simulink model "main"  (R2024b)
settings: Solver=FixedStepAuto  StartTime=0.0  StopTime=5  FixedStep=Ts  RelTol=1e-3
values from neighbouring files (symbols this model uses):
  v0 = 30    [main_data_vehicle.m]
settings Model: Creator=marti  LastModifiedBy=marti

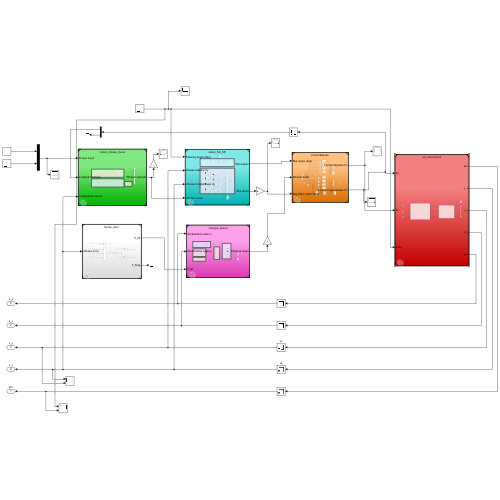
[thumbnail: Simulink's stored preview of the top-level diagram]
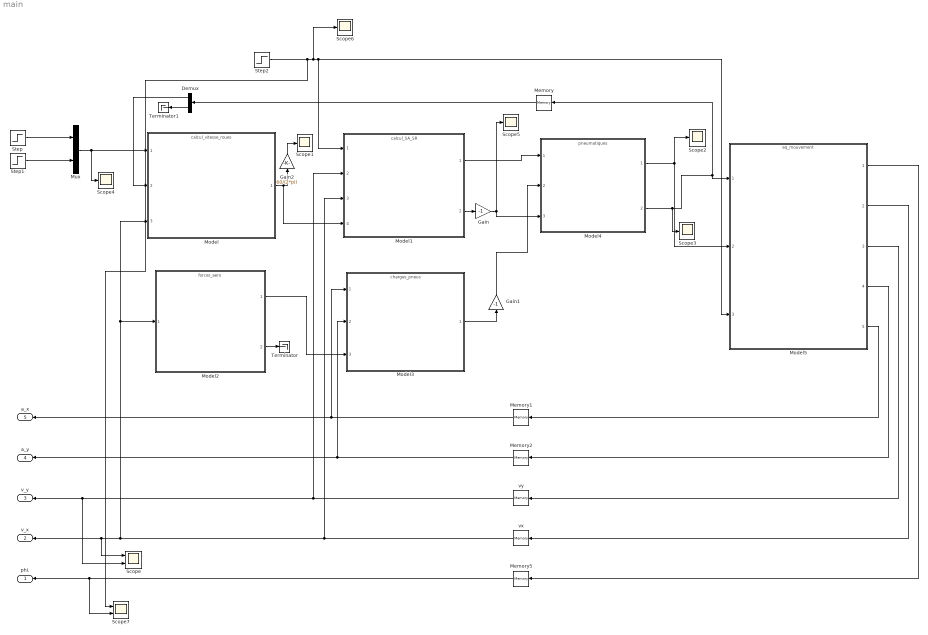
== system main ==
  Demux : Demux  Outputs=2
  Gain : Gain  Gain=-1
  Gain1 : Gain  Gain=-1
  Gain2 : Gain  Gain=60/(2*pi)
  Memory : Memory  InitialCondition=[0 0 0 0]
  Memory1 : Memory
  Memory2 : Memory
  Memory5 : Memory
  Model : ModelReference  ModelNameDialog=calcul_vitesse_roues.slx  SimulationMode=Normal  ModelReferenceVersion=1.19
  Model1 : ModelReference  ModelNameDialog=calcul_SA_SR.slx  SimulationMode=Normal  ModelReferenceVersion=1.19
  Model2 : ModelReference  ModelNameDialog=forces_aero.slx  SimulationMode=Normal  ModelReferenceVersion=1.4
  Model3 : ModelReference  ModelNameDialog=charges_pneus.slx  SimulationMode=Normal  ModelReferenceVersion=1.16
  Model4 : ModelReference  ModelNameDialog=pneumatiques.slx  SimulationMode=Normal  ModelReferenceVersion=1.15
  Model5 : ModelReference  ModelNameDialog=eq_mouvement.slx  SimulationMode=Normal  ModelReferenceVersion=1.6
  Mux : Mux  Inputs=2
  Scope : Scope  NumInputPorts=2
  Scope{1..6} (6 alike) : Scope
  Scope7 : Scope  NumInputPorts=2
  Step : Step  Time=0  After=100  SampleTime=0
  Step1 : Step  Time=0  After=300  SampleTime=0
  Step2 : Step  Time=0  After=0  SampleTime=0
  Terminator : Terminator
  Terminator1 : Terminator
  vx : Memory  InitialCondition=v0
  vy : Memory
  phi. : Outport
  v_x : Outport  Port=2
  v_y : Outport  Port=3
  a_y : Outport  Port=4
  a_x : Outport  Port=5
  wires:
  Model2/1 -> Model3/3
  Model2/2 -> Terminator/1
  Model/1 -> Model1/4, Gain2/1
  Model4/1 -> Scope2/1, Model5/2
  Model4/2 -> Scope3/1, Memory/1, Model5/1
  Model5/1 -> Memory5/1
  Model5/3 -> vy/1
  Model5/4 -> Memory2/1
  Model5/5 -> Memory1/1
  Model5/2 -> vx/1
  Step2/1 -> Scope7/1, Scope6/1, Model5/3, Model1/1
  Mux/1 -> Scope4/1, Model/1
  Memory/1 -> Demux/1
  Demux/1 -> Model/2
  Demux/2 -> Terminator1/1
  Memory1/1 -> Model3/1, a_x/1
  Memory2/1 -> Model3/2, a_y/1
  vy/1 -> Model1/2, Scope/2, v_y/1
  vx/1 -> Model1/3, Model/3, Model2/1, Scope/1, v_x/1
  Memory5/1 -> Scope7/2, phi./1
  Model3/1 -> Gain1/1
  Model1/2 -> Gain/1
  Model1/1 -> Model4/1
  Gain2/1 -> Scope1/1
  Step/1 -> Mux/1
  Step1/1 -> Mux/2
  Gain/1 -> Model4/3, Scope5/1
  Gain1/1 -> Model4/2
